simulink model "FPGADataCapture_model"  (R2019b)
settings: Solver=VariableStepAuto  StartTime=0.0  StopTime=1  RelTol=1e-3
libraries: commsink2 x1, hdlverifier_fpga_reader x1
settings Model: Creator=tcollins  LastModifiedBy=bhisma
settings DataIOCC: ReturnWorkspaceOutputs=off
settings DebuggingCC: ArithmeticOperatorsInVariantConditions=warning
settings SFSimCC: SimUseLocalCustomCode=off  CustomCodeUndefinedFunction=UseInterfaceOnly
settings RTWCC: RTWUseLocalCustomCode=off

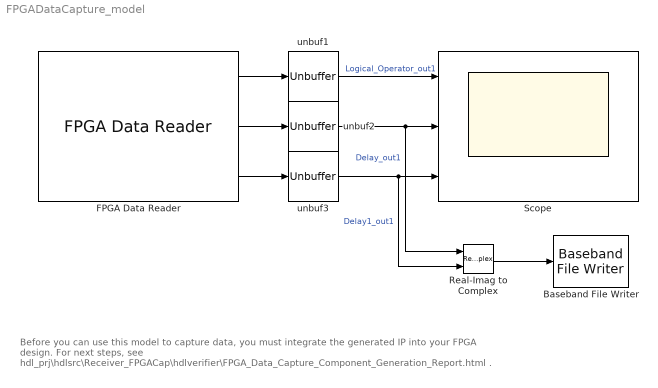
== system FPGADataCapture_model ==
  note: Before you can use this model to capture data, you must integrate the generated IP into your FPGA design.
      | For next steps, see hdl_prj\hdlsrc\Receiver_FPGACap\hdlverifier\FPGA_Data_Capture_Component_Generation_Report.html .
  Baseband File Writer : commsink2/Baseband File Writer  Filename=CRCErrorData.bb  CenterFrequency=1e9  Metadata=struct()  NumSamplesToWrite=inf  SimulateUsing=Code generation
      settings: SourceProductName=Communications Toolbox  SourceProductBaseCode=CM
  FPGA Data Reader : hdlverifier_fpga_reader/FPGA Data Reader  SampleTime=1  FPGAVendor=Xilinx  SamplesPerFrame=32768  TriggerPosition=0  TimeOut=10  TriggerConditionStr="[true,\"High\",false,\"0\",false,\"0\",\"or\"]"  DataTypeStr="[\"boolean\",\"int16\",\"int16\"]"  BitWidth="[1  16  16]"  SignalNames={'Logical_Operator_out1','Delay_out1','Delay1_out1'}  IsSignalTrigger="[1  1  1]"  IsSignalData="[1  1  1]"  JTAGCableName=auto  JTAGChainPosition=0  IRLengthBefore=0  IRLengthAfter=0  TckFrequency=15
      settings: SourceProductName=HDL Verifier Support Package for Xilinx FPGA Boards  SourceProductBaseCode=HDLCVXILINX
  Real-Imag to Complex : RealImagToComplex
  Scope : Scope  NumInputPorts=3
  unbuf1 : Unbuffer
  unbuf2 : Unbuffer
  unbuf3 : Unbuffer
  wires:
  FPGA Data Reader/1 -> unbuf1/1
  unbuf1/1 -> Scope/1  "Logical_Operator_out1"
  FPGA Data Reader/2 -> unbuf2/1
  unbuf2/1 -> Real-Imag to Complex/1, Scope/2  "Delay_out1"
  FPGA Data Reader/3 -> unbuf3/1
  unbuf3/1 -> Real-Imag to Complex/2, Scope/3  "Delay1_out1"
  Real-Imag to Complex/1 -> Baseband File Writer/1
